simulink library "Lib_Cntrl_FirstOrderSensor_TMATS"  (R2015a)
settings: Solver=ode45  StartTime=0.0  StopTime=10.0  RelTol=1e-3
Description:
  | Thomas Modules
settings Model: Creator=jwchapm2  LastModifiedBy=jwchapm2
settings OptimizationCC: ExpressionDepthLimit=2147483647
settings DebuggingCC: UnderspecifiedInitializationDetection=Classic  MergeDetectMultiDrivingBlocksExec=none  SolverPrmCheckMsg=warning  StateNameClashWarn=warning

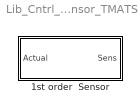
== system Lib_Cntrl_FirstOrderSensor_TMATS ==
  1st order  Sensor : Subsystem  mask(T-MATS: 1st order sensor Library Block){IC_M=0, Sen_Max_M=20000, Sen_Min_M=0, Gain_M=1, Tau_M=0.01, GN_EN_M=off, GN_NST_M=0.01, GN_C_M=1, GN_MinNoise_M=0.3, F_Gain_M=1, F_Drift_M=0}
      mask prompts: IC_M "IC_M - Sensor Initial Condition"; Sen_Max_M "Sen_Max_M - Sensor Max"; Sen_Min_M "Sen_Min_M - Sensor Min"; Gain_M "Gain_M - Sensor Gain"; Tau_M "Tau_M - Sensor Time Constant"; GN_EN_M "GN_EN_M - Noise Enabled (1 = On, 0 = Off)"; GN_NST_M "GN_NST_M - Simulation sample time"; GN_C_M "GN_C_M - Sensor scaling gain"; GN_MinNoise_M "GN_MinNoise_M - Minimum relative noise level [frac]"; F_Gain_M "F_Gain_M - Sensor Fault Gain (1 no fault)"; F_Drift_M "F_Drift_M - Sensor Drift Fault Adder (0 no fault)"
      mask help:
      | This block models a generic sensor with a first order lag.
      |
      | Additionally it may be used to simulate sensor noise, a sensor gain fault, and sensor drift fault.
      mask Help: web(which('Control_TMATS_1OS.html'),'-helpbrowser')
      mask Callback GN_EN_M: MSK_SEC_Enables_TMATS('GN_EN_M',[6 7 8],'en')

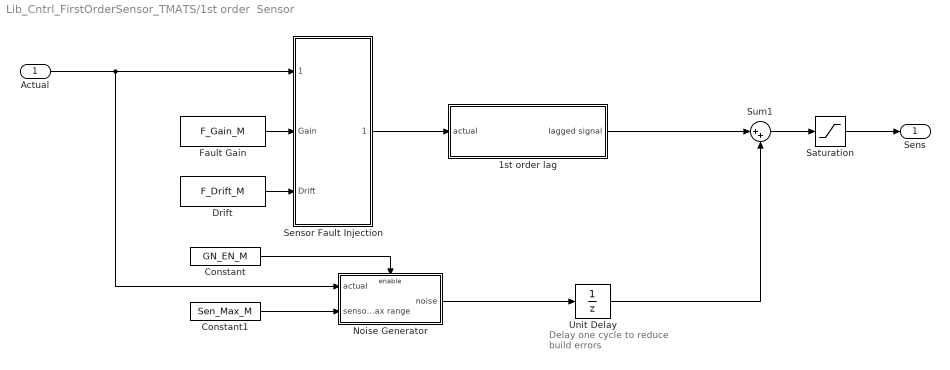
== system Lib_Cntrl_FirstOrderSensor_TMATS/1st order  Sensor ==
  note: Delay one cycle to
      | reduce build errors
  Actual : Inport
  1st order lag : Subsystem
  Constant : Constant  Value=GN_EN_M
  Constant1 : Constant  Value=Sen_Max_M
  Drift : Constant  Value=F_Drift_M
  Fault Gain : Constant  Value=F_Gain_M
  Noise Generator : Subsystem
  Saturation : Saturate  UpperLimit=Sen_Max_M  LowerLimit=Sen_Min_M
  Sensor Fault Injection : Subsystem
  Sum1 : Sum  Inputs=|++
  Unit Delay : UnitDelay  SampleTime=-1
  Sens : Outport
  wires:
  Drift/1 -> Sensor Fault Injection/3(Drift)
  Fault Gain/1 -> Sensor Fault Injection/2(Gain)
  Constant1/1 -> Noise Generator/2(sensor max range)
  Constant/1 -> Noise Generator/Enable
  Noise Generator/1(noise) -> Unit Delay/1
  Actual/1 -> Sensor Fault Injection/1(IdealSensedSig), Noise Generator/1(actual)
  Saturation/1 -> Sens/1
  1st order lag/1(lagged signal) -> Sum1/1
  Sum1/1 -> Saturation/1
  Sensor Fault Injection/1(OutSens) -> 1st order lag/1(actual)
  Unit Delay/1 -> Sum1/2

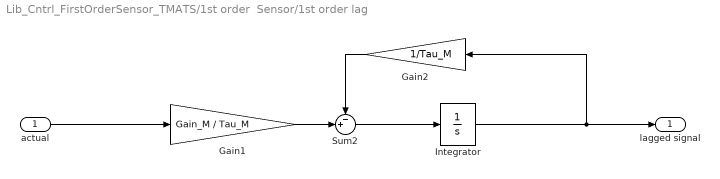
== system Lib_Cntrl_FirstOrderSensor_TMATS/1st order  Sensor/1st order lag ==
  actual : Inport
  Gain1 : Gain  Gain=Gain_M / Tau_M
  Gain2 : Gain  Gain=1/Tau_M
  Integrator : Integrator  InitialCondition=IC_M
  Sum2 : Sum  Inputs=-+|
  lagged signal : Outport
  wires:
  Integrator/1 -> lagged signal/1, Gain2/1
  actual/1 -> Gain1/1
  Sum2/1 -> Integrator/1
  Gain2/1 -> Sum2/1
  Gain1/1 -> Sum2/2

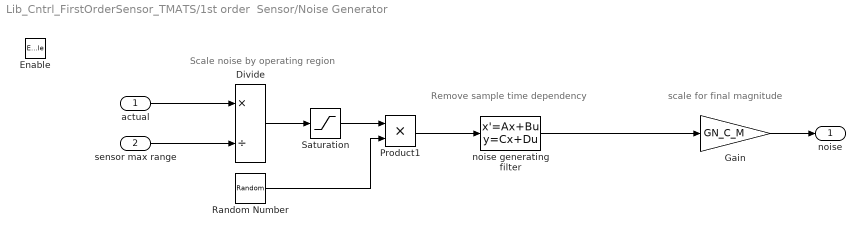
== system Lib_Cntrl_FirstOrderSensor_TMATS/1st order  Sensor/Noise Generator ==
  note: Scale noise by operating region
  note: Remove sample time dependency
  note: scale for final magnitude
  actual : Inport
  sensor max range : Inport  Port=2
  Enable : EnablePort
  Divide : Product  Inputs=*/
  Gain : Gain  Gain=GN_C_M
  Product1 : Product  RndMeth=Zero
  Random Number : RandomNumber  Seed=ceil(999999999*rand)  SampleTime=GN_NST_M
  Saturation : Saturate  UpperLimit=1  LowerLimit=GN_MinNoise_M
  noise generating filter : StateSpace  A=-1/(1-GN_NST_M/2)  D=(GN_NST_M/2)/(1-GN_NST_M/2)  X0=0
  noise : Outport
  wires:
  noise generating filter/1 -> Gain/1
  sensor max range/1 -> Divide/2
  Product1/1 -> noise generating filter/1
  actual/1 -> Divide/1
  Random Number/1 -> Product1/2
  Saturation/1 -> Product1/1
  Divide/1 -> Saturation/1
  Gain/1 -> noise/1

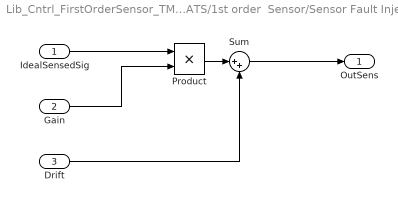
== system Lib_Cntrl_FirstOrderSensor_TMATS/1st order  Sensor/Sensor Fault Injection ==
  IdealSensedSig : Inport
  Gain : Inport  Port=2
  Drift : Inport  Port=3
  Product : Product  RndMeth=Zero
  Sum : Sum  Inputs=|++
  OutSens : Outport
  wires:
  Product/1 -> Sum/1
  Gain/1 -> Product/2
  Drift/1 -> Sum/2
  IdealSensedSig/1 -> Product/1
  Sum/1 -> OutSens/1
